simulink model "desorption_02_sim"  (R2017b)
settings: Solver=ode23tb  StartTime=0.0  StopTime=tEndSimul  MaxStep=0.1  RelTol=5e-6
values from neighbouring files (symbols this model uses):
  b_motor = 1e-3    (= 0.001)    [desorption_02.m]
  c = conversion_factors()    [desorption_02.m]
  fluid = nh3_v4    [desorption_02.m]
  h_liq_wall = 50    [desorption_02.m]
  h_reactor_air = 200    [desorption_02.m]
  h_reservoir_inner_liq = 50    [desorption_02.m]
  h_reservoir_inner_vap = 10    [desorption_02.m]
  h_reservoir_outer = 10    [desorption_02.m]
  h_vap_wall = 1e4    (= 10000)    [desorption_02.m]
  h_wall_water = 200    [desorption_02.m]
  J_motor = 0.1    [desorption_02.m]
  L_min_water = 2    [desorption_02.m]
  La_motor = 2.31e-3    (= 0.00231)    [desorption_02.m]
  Ra_motor = 2    [desorption_02.m]
  reservoir_L = 0.54    [desorption_02.m]
  rpm_init = 0    [desorption_02.m]
  rpm_ref_01 = 100*1.2    (= 120)    [desorption_02.m]
  rpm_ref_01_time = 100 * c.min_to_sec    [desorption_02.m]
  rpm_ref_02 = rpm_ref_01    (= 120)    [desorption_02.m]
  rpm_ref_02_time = rpm_ref_01_time + 3 * c.h_to_sec    [desorption_02.m]
  rpm_ref_init = 0    [desorption_02.m]
  Tamb_C = 25    [desorption_02.m]
  Tdesorp_source_C = 40    [desorption_02.m]
  Twater_in_C = 25    [desorption_02.m]
libraries: thermochemical x28, simulink x1, simulink_extras x1
settings Model: Creator=ferru  LastModifiedBy=fferrucc
settings SolverCC: ZeroCrossAlgorithm=Adaptive  AlgebraicLoopSolver=LineSearch

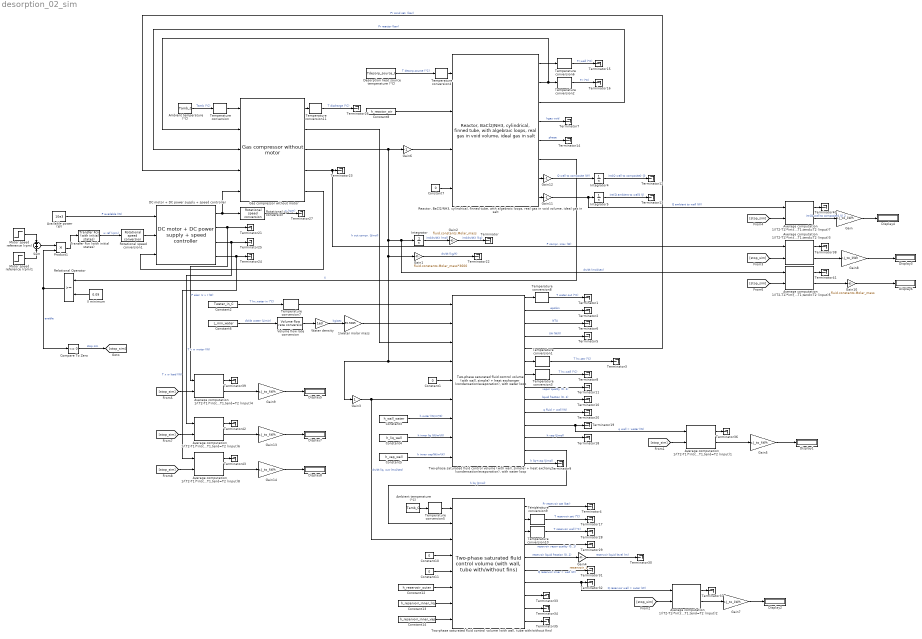
== system desorption_02_sim ==
  1/water molar mass : Gain  Gain=55.5085
  Ambient temperature (°C) : Constant  Value=Tamb_C
  "Ambient temperature (°C) " : Constant  Value=Tamb_C
  Available power (W) : Constant  Value=10e3
  Average computation 1/(T2-T1)*int{x}|t0=T1,tend=T2 (input){1..8} (8 alike) : thermochemical/Utils/Average computation 1//(T2-T1)*int{x}|t0=T1,tend=T2 (input)  T1=rpm_ref_01_time
      settings: SourceProductName=@ Thermochemical
  Compare To Zero : simulink/Logic and Bit Operations/Compare To Zero  relop=<=  OutDataTypeStr=boolean
  Constant{1,7,10..11} (4 alike) : Constant  Value=0
  Constant12 : Constant  Value=h_reservoir_outer
  Constant13 : Constant  Value=h_reservoir_inner_liq
  Constant14 : Constant  Value=h_reservoir_inner_vap
  Constant2 : Constant  Value=Twater_in_C
  Constant3 : Constant  Value=h_wall_water
  Constant4 : Constant  Value=h_liq_wall
  Constant5 : Constant  Value=h_vap_wall
  Constant6 : Constant  Value=L_min_water
  Constant8 : Constant  Value=h_reactor_air
  DC motor + DC power supply + speed controller : thermochemical/Motors/DC motor + DC power supply +  speed controller  L=La_motor  R=Ra_motor  J=J_motor  b=b_motor  Km=Km_motor  w_init_motor=rpm_init*c.rpm_to_rad_sec  PID_P=PID_P_motor  PID_I=PID_I_motor  PID_D=PID_D_motor  V_max=Vmax_motor
      settings: SourceProductName=@ Thermochemical
  Desorption heat source temperature (°C) : Constant  Value=Tdesorp_source_C
  Display{1..8} (8 alike) : Display
  Gain{,5,7..9,13..14} (7 alike) : Gain  Gain=c.J_to_kWh
  Gain1 : Gain  Gain=fluid.constants.Molar_mass*3600
  Gain10 : Gain  Gain=fluid.constants.Molar_mass
  Gain11 : Gain  Gain=-1
  Gain12 : Gain  Gain=-1
  Gain2 : Gain  Gain=fluid.constants.Molar_mass
  Gain3 : Gain
  Gain4 : Gain  Gain=reservoir_L
  Gain6 : Gain  Gain=-1
  Gas compressor without motor : thermochemical/Compression/Gas compressor without motor  fluid=fluid  eta_IS=eta_IS  CL=CL  eta_mech=eta_mech  dVswept_m3_h=dVswept_m3_h  dVswept_rmp=dVswept_rmp
      settings: SourceProductName=@ Thermochemical
  Integrator : Integrator
  Integrator4 : Integrator
  Integrator5 : Integrator
  Motor speed reference (rpm) : Step  Time=rpm_ref_01_time  Before=rpm_ref_init  After=rpm_ref_01  SampleTime=0
  Motor speed reference (rpm)1 : Step  Time=rpm_ref_02_time  After=rpm_ref_02-rpm_ref_01  SampleTime=0
  Product1 : Product
  "Reactor, BaCl2/NH3, cylindrical, finned tube, with algebraic loops, real gas in void volume, ideal gas in salt" : thermochemical/Reactors/Reactor, BaCl2//NH3, with algebraic loops, real gas in void volume, ideal gas in salt/Reactor, BaCl2//NH3, cylindrical, finned tube, with algebraic loops, real gas in void volume, ideal gas in salt
      link override "Reactor, BaCl2//NH3, cylindrical, no walls, with algebraic loops, real gas in void volume, ideal gas in salt": tao_salt=param.tao_salt  rho_composite=param.rho_composite  K_cin=K_cin  fluid=fluid  Lr=param.Lr  Lr_total=param.Lr_total  Dr=param.D  Ddiff=param.Ddiff  Tr_init=param.Tr_init  X_init=param.X_init
      link override "Wall, tube with//without fins": L_m=param.Lr_total  OD_mm=OD_mm  e_mm=thickness_mm  Tinit=Treactor_wall_init  height_fin_mm=0  thickness_fin_mm=0  pitch_fin_mm=0  material_fin=Aluminum 1100  cp_fin=905.9  rho_fin=2658  lambda_fin=211.8
      settings: SourceProductName=@ Thermochemical
  Relational Operator : RelationalOperator  OutDataTypeStr=boolean  RndMeth=Simplest
  Rotational speed conversion : thermochemical/Conversions/Rotational speed conversion  sel=rad/sec --> rpm
      settings: SourceProductName=@ Thermochemical
  Rotational speed conversion1 : thermochemical/Conversions/Rotational speed conversion  sel=rpm --> rad/sec
      settings: SourceProductName=@ Thermochemical
  Sum : Sum
  Temperature conversion{,4..5,7} (4 alike) : thermochemical/Conversions/Temperature conversion  sel=°C --> K
      settings: SourceProductName=@ Thermochemical
  Temperature conversion{1..3,6,8..11} (8 alike) : thermochemical/Conversions/Temperature conversion  sel=K --> °C
      settings: SourceProductName=@ Thermochemical
  Terminator{,1..43} (44 alike) : Terminator
  Transfer Fcn (with initial states) : simulink_extras/Additional Linear/Transfer Fcn (with initial states)  N=[1]  D="conv([1.5  1],[1.5  1])"  X0=rpm_ref_01
  "Two-phase saturated fluid control volume (with wall, tube with/without fins)" : thermochemical/Control volumes/Two-phase saturated fluid control volume (with wall, tube with//without fins)
      link override Two-phase saturated fluid control volume (without walls): N_init=reservoir_Ninit  T_init=reservoir_Tinit  V=reservoir_V
      link override "Wall, tube with//without fins": L_m=reservoir_L  OD_mm=reservoir_OD_mm  e_mm=reservoir_thickness_mm  material_tube=Stainless steel AISI316  cp_tube=490.8  rho_tube=8023
      settings: SourceProductName=@ Thermochemical
  "Two-phase saturated fluid control volume (with wall, simple) + heat exchanger (condensation/evaporation), with water loop" : thermochemical/Control volumes/Two-phase saturated fluid control volume (with wall, simple) + heat exchanger (condensation//evaporation), with water loop
      link override "Two-phase saturated fluid control volume (with wall, simple)/Two-phase saturated fluid control volume (without walls)": N_init=Nhx_init  T_init=Thx_init  V=Vhx
      link override "Two-phase saturated fluid control volume (with wall, simple)/Wall, simple, h as inputs": material=Stainless steel AISI316  cp=490.8  rho=8023  s=Shx_m2  e_mm=thickness_hx_mm  mass=2.2529
      settings: SourceProductName=@ Thermochemical
  Volume flow rate conversion : thermochemical/Conversions/Volume flow rate conversion  sel=L/min --> m3/sec
      settings: SourceProductName=@ Thermochemical
  Water density : Gain  Gain=1e3
  X minimum : Constant  Value=0.09
  wires:
  Integrator/1 -> Gain2/1  "int{dn/dt} (mol)"
  Temperature conversion2/1 -> Terminator16/1  "Tr (°C)"
  Temperature conversion6/1 -> Terminator15/1  "Tr,wall (°C)"
  "Reactor, BaCl2/NH3, cylindrical, finned tube, with algebraic loops, real gas in void volume, ideal gas in salt"/4 -> Terminator7/1  "hgas void"
  "Reactor, BaCl2/NH3, cylindrical, finned tube, with algebraic loops, real gas in void volume, ideal gas in salt"/5 -> Terminator14/1  "phase"
  "Reactor, BaCl2/NH3, cylindrical, finned tube, with algebraic loops, real gas in void volume, ideal gas in salt"/2 -> Temperature conversion2/1, Gas compressor without motor/2
  "Reactor, BaCl2/NH3, cylindrical, finned tube, with algebraic loops, real gas in void volume, ideal gas in salt"/6 -> Relational Operator/1  "X"
  "Reactor, BaCl2/NH3, cylindrical, finned tube, with algebraic loops, real gas in void volume, ideal gas in salt"/3 -> Gas compressor without motor/3  "Pr reactor (bar)"
  "Reactor, BaCl2/NH3, cylindrical, finned tube, with algebraic loops, real gas in void volume, ideal gas in salt"/1 -> Temperature conversion6/1
  Gain11/1 -> "Average computation 1/(T2-T1)*int{x}|t0=T1,tend=T2 (input)7"/1, Integrator5/1  "Q ambient to wall (W)"
  "Reactor, BaCl2/NH3, cylindrical, finned tube, with algebraic loops, real gas in void volume, ideal gas in salt"/8 -> Gain11/1
  Integrator4/1 -> Terminator12/1  "int{Q wall to composite} (J)"
  Gain12/1 -> Integrator4/1  "Q wall to composite (W)"
  Integrator5/1 -> Terminator13/1  "int{Q ambient to wall} (J)"
  "Reactor, BaCl2/NH3, cylindrical, finned tube, with algebraic loops, real gas in void volume, ideal gas in salt"/7 -> Gain12/1
  "Two-phase saturated fluid control volume (with wall, simple) + heat exchanger (condensation/evaporation), with water loop"/10 -> Terminator20/1  "q fluid > wall (W)"
  "Two-phase saturated fluid control volume (with wall, simple) + heat exchanger (condensation/evaporation), with water loop"/9 -> Terminator10/1  "liquid fraction (0..1)"
  Water density/1 -> 1/water molar mass/1  "kg/sec"
  Temperature conversion3/1 -> Terminator8/1  "T hx,wall (°C)"
  "Two-phase saturated fluid control volume (with wall, simple) + heat exchanger (condensation/evaporation), with water loop"/11 -> "Average computation 1/(T2-T1)*int{x}|t0=T1,tend=T2 (input)1"/1, Terminator19/1  "q wall > water (W)"
  Constant2/1 -> Temperature conversion7/1  "T hx,water in (°C)"
  "Two-phase saturated fluid control volume (with wall, simple) + heat exchanger (condensation/evaporation), with water loop"/2 -> Terminator2/1  "epsilon"
  "Two-phase saturated fluid control volume (with wall, simple) + heat exchanger (condensation/evaporation), with water loop"/4 -> Terminator5/1  "UA (W/K)"
  "Two-phase saturated fluid control volume (with wall, simple) + heat exchanger (condensation/evaporation), with water loop"/12 -> Terminator18/1  "h vap (J/mol)"
  "Two-phase saturated fluid control volume (with wall, simple) + heat exchanger (condensation/evaporation), with water loop"/1 -> Temperature conversion8/1
  "Two-phase saturated fluid control volume (with wall, simple) + heat exchanger (condensation/evaporation), with water loop"/13 -> "Two-phase saturated fluid control volume (with wall, tube with/without fins)"/2  "h liq (J/mol)"
  Volume flow rate conversion/1 -> Water density/1
  "Two-phase saturated fluid control volume (with wall, simple) + heat exchanger (condensation/evaporation), with water loop"/3 -> Terminator6/1  "NTU"
  Temperature conversion8/1 -> Terminator1/1  "T water out (°C)"
  "Two-phase saturated fluid control volume (with wall, simple) + heat exchanger (condensation/evaporation), with water loop"/6 -> Temperature conversion1/1
  "Two-phase saturated fluid control volume (with wall, simple) + heat exchanger (condensation/evaporation), with water loop"/14 -> Terminator9/1  "h liq+vap (J/mol)"
  Constant4/1 -> "Two-phase saturated fluid control volume (with wall, simple) + heat exchanger (condensation/evaporation), with water loop"/8  "h inner liq (W/m²/K)"
  Constant5/1 -> "Two-phase saturated fluid control volume (with wall, simple) + heat exchanger (condensation/evaporation), with water loop"/9  "h inner vap(W/m²/K)"
  "Two-phase saturated fluid control volume (with wall, simple) + heat exchanger (condensation/evaporation), with water loop"/7 -> Temperature conversion3/1
  Constant3/1 -> "Two-phase saturated fluid control volume (with wall, simple) + heat exchanger (condensation/evaporation), with water loop"/7  "h outer (W/m²/K)"
  Temperature conversion1/1 -> Terminator3/1  "T hx,sat (°C)"
  "Two-phase saturated fluid control volume (with wall, simple) + heat exchanger (condensation/evaporation), with water loop"/8 -> Terminator11/1  "vapor quality (0..1)"
  Gain3/1 -> "Two-phase saturated fluid control volume (with wall, tube with/without fins)"/3, "Two-phase saturated fluid control volume (with wall, simple) + heat exchanger (condensation/evaporation), with water loop"/6  "dn/dt liq, out (mol/sec)"
  Temperature conversion7/1 -> "Two-phase saturated fluid control volume (with wall, simple) + heat exchanger (condensation/evaporation), with water loop"/1
  Gas compressor without motor/4 -> "Average computation 1/(T2-T1)*int{x}|t0=T1,tend=T2 (input)3"/1, Terminator23/1  "P compr. irrev (W)"
  DC motor + DC power supply + speed controller/2 -> "Average computation 1/(T2-T1)*int{x}|t0=T1,tend=T2 (input)4"/1, Terminator21/1  "P elec: U x I (W)"
  Rotational speed conversion1/1 -> DC motor + DC power supply + speed controller/2
  DC motor + DC power supply + speed controller/3 -> "Average computation 1/(T2-T1)*int{x}|t0=T1,tend=T2 (input)6"/1, Terminator25/1  "T x w motor (W)"
  Motor speed reference (rpm)/1 -> Sum/1
  Temperature conversion11/1 -> Terminator26/1  "T discharge (°C)"
  Rotational speed conversion/1 -> Terminator27/1  "w (rpm)"
  Temperature conversion/1 -> Gas compressor without motor/1
  Gas compressor without motor/1 -> Temperature conversion11/1
  Gas compressor without motor/5 -> DC motor + DC power supply + speed controller/3
  Ambient temperature (°C)/1 -> Temperature conversion/1  "Tamb (°C)"
  Available power (W)/1 -> DC motor + DC power supply + speed controller/1  "P available (W)"
  DC motor + DC power supply + speed controller/1 -> Gas compressor without motor/5, Rotational speed conversion/1
  DC motor + DC power supply + speed controller/4 -> "Average computation 1/(T2-T1)*int{x}|t0=T1,tend=T2 (input)8"/1, Terminator24/1  "T x w load (W)"
  Transfer Fcn (with initial states)/1 -> Rotational speed conversion1/1  "w ref (rpm)"
  Gas compressor without motor/3 -> "Average computation 1/(T2-T1)*int{x}|t0=T1,tend=T2 (input)5"/1, Integrator/1, Gain1/1, Gain3/1, "Two-phase saturated fluid control volume (with wall, simple) + heat exchanger (condensation/evaporation), with water loop"/4, Gain6/1  "dn/dt (mol/sec)"
  Constant7/1 -> "Reactor, BaCl2/NH3, cylindrical, finned tube, with algebraic loops, real gas in void volume, ideal gas in salt"/4
  Gain6/1 -> "Reactor, BaCl2/NH3, cylindrical, finned tube, with algebraic loops, real gas in void volume, ideal gas in salt"/3
  Gas compressor without motor/2 -> "Two-phase saturated fluid control volume (with wall, simple) + heat exchanger (condensation/evaporation), with water loop"/3  "h out compr. (J/mol)"
  Constant1/1 -> "Two-phase saturated fluid control volume (with wall, simple) + heat exchanger (condensation/evaporation), with water loop"/5
  Constant6/1 -> Volume flow rate conversion/1  "dV/dt water (L/min)"
  1/water molar mass/1 -> "Two-phase saturated fluid control volume (with wall, simple) + heat exchanger (condensation/evaporation), with water loop"/2
  Desorption heat source temperature (°C)/1 -> Temperature conversion4/1  "T desorp,source (°C)"
  Temperature conversion4/1 -> "Reactor, BaCl2/NH3, cylindrical, finned tube, with algebraic loops, real gas in void volume, ideal gas in salt"/1
  Constant8/1 -> "Reactor, BaCl2/NH3, cylindrical, finned tube, with algebraic loops, real gas in void volume, ideal gas in salt"/2
  Motor speed reference (rpm)1/1 -> Sum/2
  Sum/1 -> Product1/1
  Gain1/1 -> Terminator22/1  "dn/dt (kg/h)"
  Gain2/1 -> Terminator/1  "int{dn/dt} (kg)"
  "Ambient temperature (°C) "/1 -> Temperature conversion5/1
  Temperature conversion5/1 -> "Two-phase saturated fluid control volume (with wall, tube with/without fins)"/1
  Constant10/1 -> "Two-phase saturated fluid control volume (with wall, tube with/without fins)"/4
  Constant11/1 -> "Two-phase saturated fluid control volume (with wall, tube with/without fins)"/5
  Constant12/1 -> "Two-phase saturated fluid control volume (with wall, tube with/without fins)"/6
  Constant13/1 -> "Two-phase saturated fluid control volume (with wall, tube with/without fins)"/7
  Constant14/1 -> "Two-phase saturated fluid control volume (with wall, tube with/without fins)"/8
  "Two-phase saturated fluid control volume (with wall, tube with/without fins)"/1 -> Terminator4/1  "Pr reservoir sat (bar)"
  Temperature conversion9/1 -> Terminator17/1  "T reservoir sat (°C)"
  "Two-phase saturated fluid control volume (with wall, tube with/without fins)"/3 -> Temperature conversion10/1
  "Two-phase saturated fluid control volume (with wall, tube with/without fins)"/5 -> Gain4/1  "reservoir liquid fraction (0..1)"
  "Two-phase saturated fluid control volume (with wall, tube with/without fins)"/6 -> Terminator31/1  "Q reservoir inner > wall (W)"
  "Two-phase saturated fluid control volume (with wall, tube with/without fins)"/7 -> "Average computation 1/(T2-T1)*int{x}|t0=T1,tend=T2 (input)2"/1, Terminator32/1  "Q reservoir wall > outer (W)"
  "Two-phase saturated fluid control volume (with wall, tube with/without fins)"/8 -> Terminator33/1
  "Two-phase saturated fluid control volume (with wall, tube with/without fins)"/9 -> Terminator34/1
  "Two-phase saturated fluid control volume (with wall, tube with/without fins)"/10 -> Terminator35/1
  "Two-phase saturated fluid control volume (with wall, tube with/without fins)"/2 -> Temperature conversion9/1
  Temperature conversion10/1 -> Terminator28/1  "T reservoir wall (°C)"
  "Two-phase saturated fluid control volume (with wall, tube with/without fins)"/4 -> Terminator29/1  "reservoir vapor quality (0..1)"
  Gain4/1 -> Terminator30/1  "reservoir liquid level (m)"
  Product1/1 -> Transfer Fcn (with initial states)/1
  X minimum/1 -> Relational Operator/2
  Relational Operator/1 -> Compare To Zero/1, Product1/2  "enable"
  "Two-phase saturated fluid control volume (with wall, simple) + heat exchanger (condensation/evaporation), with water loop"/5 -> Gas compressor without motor/4  "Pr cond sat. (bar)"
  "Average computation 1/(T2-T1)*int{x}|t0=T1,tend=T2 (input)7"/1 -> Terminator40/1
  [stop_sim] -> "Average computation 1/(T2-T1)*int{x}|t0=T1,tend=T2 (input)7"/2
  "Average computation 1/(T2-T1)*int{x}|t0=T1,tend=T2 (input)7"/2 -> Gain/1  "int{Q wall to composite} (J) 2"
  Compare To Zero/1 -> [stop_sim]  "stop sim"
  Gain/1 -> Display4/1
  Gain5/1 -> Display1/1
  "Average computation 1/(T2-T1)*int{x}|t0=T1,tend=T2 (input)1"/2 -> Gain5/1
  [stop_sim] -> "Average computation 1/(T2-T1)*int{x}|t0=T1,tend=T2 (input)1"/2
  "Average computation 1/(T2-T1)*int{x}|t0=T1,tend=T2 (input)1"/1 -> Terminator36/1
  "Average computation 1/(T2-T1)*int{x}|t0=T1,tend=T2 (input)2"/1 -> Terminator37/1
  [stop_sim] -> "Average computation 1/(T2-T1)*int{x}|t0=T1,tend=T2 (input)2"/2
  "Average computation 1/(T2-T1)*int{x}|t0=T1,tend=T2 (input)2"/2 -> Gain7/1
  Gain7/1 -> Display2/1
  "Average computation 1/(T2-T1)*int{x}|t0=T1,tend=T2 (input)3"/1 -> Terminator38/1
  [stop_sim] -> "Average computation 1/(T2-T1)*int{x}|t0=T1,tend=T2 (input)3"/2
  "Average computation 1/(T2-T1)*int{x}|t0=T1,tend=T2 (input)3"/2 -> Gain8/1
  Gain8/1 -> Display3/1
  Gain9/1 -> Display5/1
  "Average computation 1/(T2-T1)*int{x}|t0=T1,tend=T2 (input)4"/2 -> Gain9/1
  [stop_sim] -> "Average computation 1/(T2-T1)*int{x}|t0=T1,tend=T2 (input)4"/2
  "Average computation 1/(T2-T1)*int{x}|t0=T1,tend=T2 (input)4"/1 -> Terminator39/1
  "Average computation 1/(T2-T1)*int{x}|t0=T1,tend=T2 (input)5"/1 -> Terminator41/1
  [stop_sim] -> "Average computation 1/(T2-T1)*int{x}|t0=T1,tend=T2 (input)5"/2
  "Average computation 1/(T2-T1)*int{x}|t0=T1,tend=T2 (input)5"/2 -> Gain10/1
  Gain10/1 -> Display6/1
  "Average computation 1/(T2-T1)*int{x}|t0=T1,tend=T2 (input)6"/1 -> Terminator42/1
  [stop_sim] -> "Average computation 1/(T2-T1)*int{x}|t0=T1,tend=T2 (input)6"/2
  "Average computation 1/(T2-T1)*int{x}|t0=T1,tend=T2 (input)6"/2 -> Gain13/1
  Gain13/1 -> Display7/1
  Gain14/1 -> Display8/1
  "Average computation 1/(T2-T1)*int{x}|t0=T1,tend=T2 (input)8"/2 -> Gain14/1
  [stop_sim] -> "Average computation 1/(T2-T1)*int{x}|t0=T1,tend=T2 (input)8"/2
  "Average computation 1/(T2-T1)*int{x}|t0=T1,tend=T2 (input)8"/1 -> Terminator43/1
